simulink model "ad9364_sim"  (R2017b)
settings: Solver=ode45  StartTime=0.0  StopTime=Inf  RelTol=1e-3  EnableMultiTasking=on
libraries: dspsrcs4 x2, simulink x2
settings Model: Creator=ACozma  LastModifiedBy=ACozma
settings DataIOCC: LimitDataPoints=on  SaveFormat=Array
settings OptimizationCC: LifeSpan=inf
settings DebuggingCC: UnderspecifiedInitializationDetection=Classic  MergeDetectMultiDrivingBlocksExec=none  SolverPrmCheckMsg=warning  SFUnexpectedBacktrackingDiag=warning  SFNoUnconditionalDefaultTransitionDiag=warning  SFExecutionAtInitializationDiag=none
settings HardwareCC: ProdBitPerPointer=32  ProdBitPerSizeT=32  ProdBitPerPtrDiffT=32  ProdLargestAtomicFloat=None  ProdIntDivRoundTo=Undefined  ProdEndianess=Unspecified  ProdWordSize=32  ProdHWDeviceType=32-bit Generic
settings ModelReferenceCC: PropagateSignalLabelsOutOfModel=off
settings CodeAppCC: StateflowObjectComments=on
settings GRTTargetCC: TargetLangStandard=C89/C90 (ANSI)  GeneratePreprocessorConditionals=Disable all
settings ConfigComp: CovMetricSettings=dw  CovHtmlReporting=on  CovSaveCumulativeToWorkspaceVar=on  CovSaveSingleToWorkspaceVar=on  CovExternalEMLEnable=off  CovSFcnEnable=off

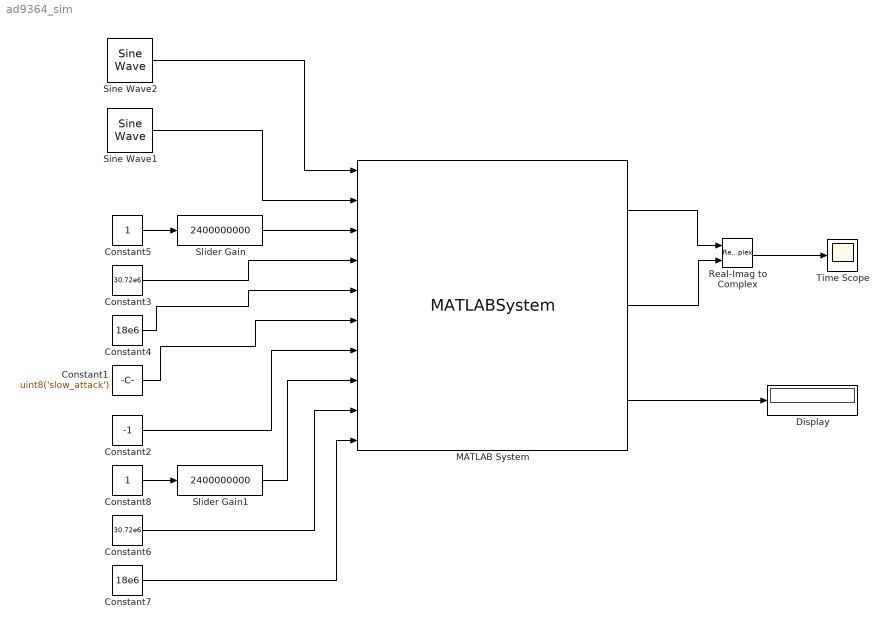
== system ad9364_sim ==
  Constant1 : Constant  Value=uint8('slow_attack')  SampleTime=-1
  Constant2 : Constant  Value=-1  SampleTime=-1
  Constant3 : Constant  Value=30.72e6  SampleTime=-1
  Constant4 : Constant  Value=18e6  SampleTime=-1
  Constant5 : Constant  SampleTime=-1
  Constant6 : Constant  Value=30.72e6  SampleTime=-1
  Constant7 : Constant  Value=18e6  SampleTime=-1
  Constant8 : Constant  SampleTime=-1
  Display : Display
  MATLAB System : MATLABSystem  DialogController=sysobjdialog.BlockDynDialog  System=iio_sys_obj  ip_address=192.168.3.2  dev_name=ad9364  in_ch_no=2  in_ch_size=32768  out_ch_no=2  out_ch_size=8192  SimulateUsing=Interpreted execution
      mask Type: iio_sys_obj
      mask Display:
      | disp('ad9364');
      | port_label('input',1,'DATA_IN1');
      | port_label('input',2,'DATA_IN2');
      | port_label('input',3,'RX_LO_FREQ');
      | port_label('input',4,'RX_SAMPLING_FREQ');
      | port_label('input',5,'RX_RF_BANDWIDTH');
      | port_label('input',6,'RX_GAIN_MODE');
      | port_label('input',7,'RX_GAIN');
      | port_label('input',8,'TX_LO_FREQ');
      | port_label('input',9,'TX_SAMPLING_FREQ');
      | port_label('input',10,'TX_RF_BANDWIDTH');
      | port_label('output',1,'DATA_OUT1');
      | port_label('output',2,'DATA_OUT2');
      | port_label('output',3,'RX_RSSI');
  Real-Imag to Complex : RealImagToComplex
  Sine Wave1 : dspsrcs4/Sine Wave  Amplitude=32768  Frequency=100  Phase=pi/2  SampleMode=Discrete  OutComplex=Real  CompMethod=Trigonometric fcn  TableSize=Speed  SampleTime=1/10000  SamplesPerFrame=32768  ResetState=Catch up to simulation time  OutputFrames=on  dataType=double  wordLen=16  udDataType=sfix(16)  fracBitsMode=Best precision  numFracBits=15  OutDataTypeStr=double  LastOutDataTypeStr=double
  Sine Wave2 : dspsrcs4/Sine Wave  Amplitude=32768  Frequency=100  Phase=0  SampleMode=Discrete  OutComplex=Real  CompMethod=Trigonometric fcn  TableSize=Speed  SampleTime=1/10000  SamplesPerFrame=32768  ResetState=Catch up to simulation time  OutputFrames=on  dataType=double  wordLen=16  udDataType=sfix(16)  fracBitsMode=Best precision  numFracBits=15  OutDataTypeStr=double  LastOutDataTypeStr=double
  Slider Gain : simulink/Math Operations/Slider Gain  gain=2400000000  low=200000  high=6000000000
  Slider Gain1 : simulink/Math Operations/Slider Gain  gain=2400000000  low=200000  high=6000000000
  Time Scope : Scope
  wires:
  Slider Gain/1 -> MATLAB System/3
  Constant3/1 -> MATLAB System/4
  Constant4/1 -> MATLAB System/5
  Constant1/1 -> MATLAB System/6
  Constant2/1 -> MATLAB System/7
  Slider Gain1/1 -> MATLAB System/8
  Constant5/1 -> Slider Gain/1
  Constant8/1 -> Slider Gain1/1
  Constant6/1 -> MATLAB System/9
  Constant7/1 -> MATLAB System/10
  MATLAB System/3 -> Display/1
  MATLAB System/1 -> Real-Imag to Complex/1
  MATLAB System/2 -> Real-Imag to Complex/2
  Sine Wave2/1 -> MATLAB System/1
  Sine Wave1/1 -> MATLAB System/2
  Real-Imag to Complex/1 -> Time Scope/1
